simulink model "PM_fnc13_TestHarness"  (R2022a)
settings: Solver=FixedStepAuto  StartTime=0.0  StopTime=inf  FixedStep=1  RelTol=1e-3
undefined symbols (not defined in the file or in its folder): cal_dchg_falling_slew_rate, cal_dchg_PL1_ini, cal_dchg_rising_slew_rate
libraries: simulink x2
settings Model: PacingRate=1.500000  Creator=306427  LastModifiedBy=306427

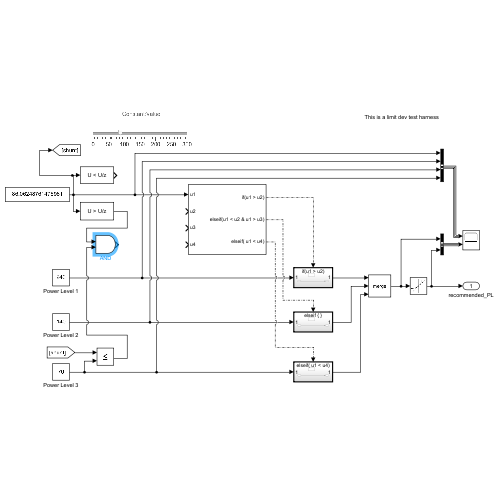
[thumbnail: Simulink's stored preview of the top-level diagram]
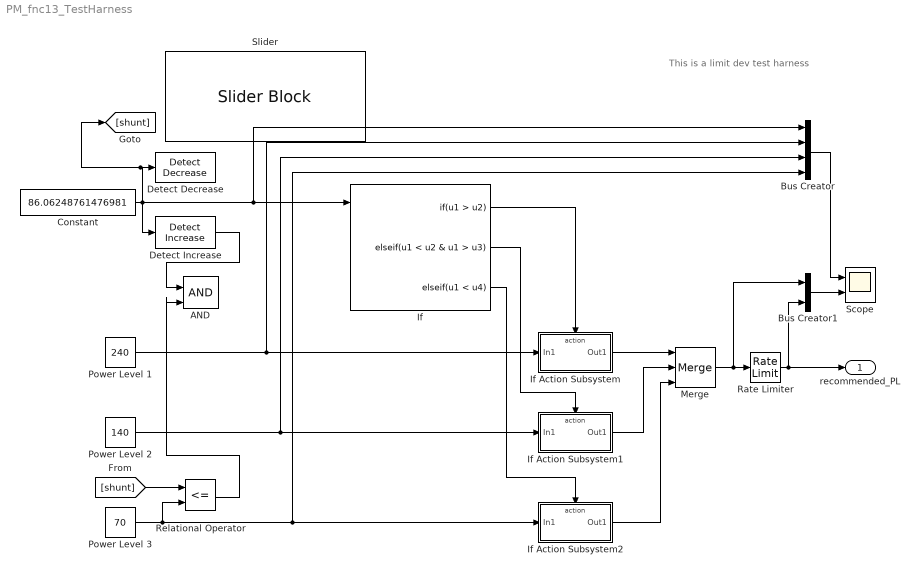
== system PM_fnc13_TestHarness ==
  note: This is a limit dev test harness
  AND : Logic  IconShape=distinctive  AllPortsSameDT=off  OutDataTypeStr=boolean
  Bus Creator : BusCreator  Inputs=4
  Bus Creator1 : BusCreator  Inputs=2
  Constant : Constant  Value=86.06248761476981
  Detect Decrease : simulink/Logic and Bit Operations/Detect Decrease  vinit=0.0  OutDataTypeStr=boolean
  Detect Increase : simulink/Logic and Bit Operations/Detect Increase  vinit=0.0  OutDataTypeStr=boolean
  If : If  NumInputs=4  IfExpression=u1 > u2  ElseIfExpressions=u1 < u2 & u1 > u3, u1 < u4  ShowElse=off
  If Action Subsystem : Subsystem  TreatAsAtomicUnit=on
  If Action Subsystem1 : Subsystem  TreatAsAtomicUnit=on
  If Action Subsystem2 : Subsystem  TreatAsAtomicUnit=on
  Merge : Merge  Inputs=3
  Power Level 1 : Constant  Value=240
  Power Level 2 : Constant  Value=140
  Power Level 3 : Constant  Value=70
  Rate Limiter : RateLimiter  RisingSlewLimit=cal_dchg_rising_slew_rate  FallingSlewLimit=cal_dchg_falling_slew_rate  SampleTimeMode=inherited  InitialCondition=cal_dchg_PL1_ini
  Relational Operator : RelationalOperator  Operator=<=  OutDataTypeStr=boolean  RndMeth=Simplest  InputSameDT=off
  Scope : Scope  NumInputPorts=2
  Slider : SliderBlock  ScaleMax=300
  recommended_PL : Outport
  wires:
  Power Level 1/1 -> If Action Subsystem/1(In1), Bus Creator/2
  Power Level 2/1 -> If Action Subsystem1/1(In1), Bus Creator/3
  Power Level 3/1 -> Relational Operator/2, If Action Subsystem2/1(In1), Bus Creator/4
  If Action Subsystem/1(Out1) -> Merge/1
  If Action Subsystem1/1(Out1) -> Merge/2
  If Action Subsystem2/1(Out1) -> Merge/3
  Constant/1 -> Detect Increase/1, [shunt], Detect Decrease/1, Bus Creator/1, If/1
  If/1 -> If Action Subsystem/Action
  If/2 -> If Action Subsystem1/Action
  If/3 -> If Action Subsystem2/Action
  Merge/1 -> Bus Creator1/1, Rate Limiter/1
  Rate Limiter/1 -> Bus Creator1/2, recommended_PL/1
  Bus Creator/1 -> Scope/1
  Bus Creator1/1 -> Scope/2
  [shunt] -> Relational Operator/1
  Relational Operator/1 -> AND/2
  Detect Increase/1 -> AND/1

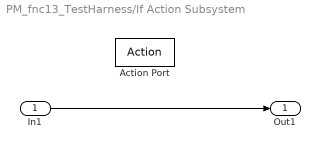
== system PM_fnc13_TestHarness/If Action Subsystem ==
  In1 : Inport
  Action Port : ActionPort  ActionPortLabel=if(u1 > u2)
  Out1 : Outport
  wires:
  In1/1 -> Out1/1

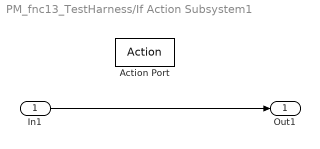
== system PM_fnc13_TestHarness/If Action Subsystem1 ==
  In1 : Inport
  Action Port : ActionPort  ActionPortLabel=elseif(u1 < u2 & u1 > u3)
  Out1 : Outport
  wires:
  In1/1 -> Out1/1

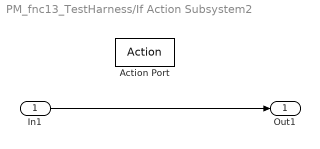
== system PM_fnc13_TestHarness/If Action Subsystem2 ==
  In1 : Inport
  Action Port : ActionPort  ActionPortLabel=elseif( u1 < u4)
  Out1 : Outport
  wires:
  In1/1 -> Out1/1
